simulink model "MATMPC_SIMULINK"  (R2017b)
settings: Solver=VariableStepAuto  StartTime=0.0  StopTime=4.0  RelTol=1e-3
values from neighbouring files (symbols this model uses):
  lb = 0*ones(nc,1)    [InitData.m]    (also in Initialization.m; Initialization_Simulink.m = 0)
  lbu = -80*ones(nu,1)    [InitData.m]    (also in InitData_ngrid.m = -inf(nu,1); Initialization.m; Initialization_Simulink.m = repmat(lbu,1,N))
  lbx = 0    [Initialization_Simulink.m]
  para = repmat(para0,1,N+1)    [InitData.m]    (also in InitData_ngrid.m = repmat(para0,1,r+1); Initialization.m; Initialization_Simulink.m)
  ref = zeros(ny,1)    [Initialization_Simulink.m]
  Ts = 0.2    [ChainofMasses_NLin.m]    (also in DiM.m = 0.01; InitData.m = settings.Ts; InitData_ngrid.m = settings.Ts; InitMemory.m = settings.Ts)
  ub = 12*ones(nc,1)    [InitData.m]    (also in Initialization.m; Initialization_Simulink.m = 0)
  ubu = 80*ones(nu,1)    [InitData.m]    (also in InitData_ngrid.m = inf(nu,1); Initialization.m; Initialization_Simulink.m = repmat(ubu,1,N))
  ubx = 0    [Initialization_Simulink.m]
  W = eye(3)    [DiM.m]    (also in Initialization_Simulink.m = diag([10 10 0.1 0.1 0.01]))
  WN = W(1:nyN,1:nyN)    [Initialization_Simulink.m]
  x0 = zeros(nx,1)    [InitData.m]    (also in Initialization.m; Initialization_Simulink.m = [0;pi;0;0])
settings Model: Creator=chen  LastModifiedBy=chen
settings RTWCC: CheckMdlBeforeBuild=Error

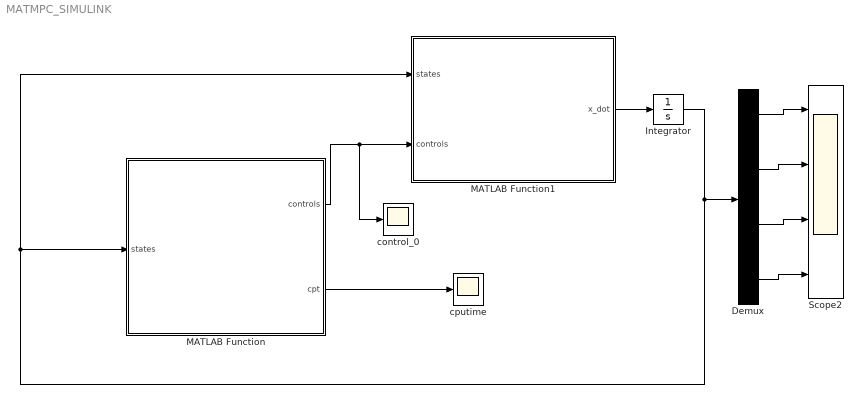
== system MATMPC_SIMULINK ==
  Demux : Demux
  Integrator : Integrator  InitialCondition=x0
  MATLAB Function : MATLAB Function  TreatAsAtomicUnit=on  SystemSampleTime=Ts
  MATLAB Function1 : MATLAB Function  TreatAsAtomicUnit=on
  Scope2 : Scope  NumInputPorts=4
  control_0 : Scope
  cputime : Scope
  wires:
  MATLAB Function/1(controls) -> control_0/1, MATLAB Function1/2(controls)
  MATLAB Function/2(cpt) -> cputime/1
  MATLAB Function1/1(x_dot) -> Integrator/1
  Integrator/1 -> Demux/1, MATLAB Function/1(states), MATLAB Function1/1(states)
  Demux/1 -> Scope2/1
  Demux/2 -> Scope2/2
  Demux/3 -> Scope2/3
  Demux/4 -> Scope2/4

== matlab function MATMPC_SIMULINK/MATLAB Function1 ==
  data: states input size=4; x_dot output size=4; controls input size=1
function x_dot  = Dynamics(states,controls)

M = 1; 
m = 0.1;
l = 0.8; 
g = 9.81;

p=states(1);
theta=states(2);
v=states(3);
omega=states(4);  
u=controls(1);

a=-m*l*sin(theta)*omega^2+m*g*cos(theta)*sin(theta)+u;
b=-m*l*cos(theta)*sin(theta)*omega^2+u*cos(theta)+(M+m)*g*sin(theta);
c=M+m-m*(cos(theta))^2;

x_dot = [v;omega;a/c;b/(l*c)];

return

== matlab function MATMPC_SIMULINK/MATLAB Function ==
  settings: updateMethod=DISCRETE
  data: states input size=4; controls output size=1; cpt output size=1; x0 parameter; lb parameter; ub parameter; lbx parameter; ubx parameter; lbu parameter; ubu parameter; W parameter; WN parameter; para parameter; ref parameter
function [controls,cpt] = NMPC_BLOCK(states, x0, lb, ub, lbx, ubx, lbu, ubu, W, WN, para, ref)

%% everything should has a fixed size

coder.extrinsic('mpc_nmpcsolver_simulink');  
coder.extrinsic('InitData');  
coder.extrinsic('InitMemory');  
%%

persistent x u lambda mu mu_x mu_u;
persistent input mem opt settings;

if isempty(x)  
    
    N=40;
    N2=5;
    Ts  = 0.05;
    Ts_st = 0.05;
    s = 2;     
    nx = 4;    
    nu = 1;   
    ny = 5;    
    nyN= 4;   
    np = 0;    
    nc = 0;    
    ncN = 0;  
    nbx = 1;
    nbu = 1;
    nbu_idx = 1;
    nbx_idx = 1;
    
    settings.N=N;
    settings.N2=N2;
    settings.Ts = Ts;
    settings.Ts_st = Ts_st;
    settings.s =s ;
    settings.nx = nx; 
    settings.nu = nu;    
    settings.ny = ny;    
    settings.nyN= nyN;    
    settings.np = np;   
    settings.nc = nc;
    settings.ncN = ncN;
    settings.nbx = nbx;
    settings.nbu = nbu;
    settings.nbx_idx = nbx_idx;
    settings.nbu_idx = nbu_idx;
    settings.model='InvertedPendulum';
    
    opt.integrator='ERK4-CASADI'; % 'ERK4','IRK3, 'ERK4-CASADI'
    opt.hessian='gauss_newton';  % 'gauss_newton'
    opt.condensing='default_full';  %'default_full','no'
    opt.qpsolver='qpoases'; %'qpoases','qore', 'quadprog', 'hpipm_sparse', 'hpipm_pcond'
    opt.hotstart='no'; %'yes','no' (only for qpoases)
    opt.shifting='yes'; % 'yes','no'
    opt.lin_obj='yes'; % 'yes','no' % if objective function is linear least square
    opt.ref_type=0; % 0-time invariant, 1-time varying(no preview), 2-time varying (preview)
   
    input.x0=x0;
    
    x=repmat(x0,1,N+1);
    input.x=x;
    
    u=zeros(nu,N);
    input.u=u;
    
    lambda = zeros(nx,N+1);
    input.lambda= lambda;
    
    if N*nc+ncN > 0
        mu = zeros(N*nc+ncN,1);
    else
        mu = 0;
    end
    input.mu= mu;
    
    mu_u = zeros(N*nu,1);
    input.mu_u= mu_u;
    
    if (N+1)*nbx > 0
        mu_x = zeros((N+1)*nbx,1);
    else
        mu_x = 0;
    end
    input.mu_x = mu_x;
    
    input.lb = lb;
    input.ub = ub;
    input.lbx = lbx;
    input.ubx = ubx;
    input.lbu = lbu;
    input.ubu = ubu;
    
    input.W=W;
    input.WN=WN;
    input.od = para;
    
    input.y = repmat(ref,1,N);
    input.yN = ref(1:nyN,1);
    
    mem.warm_start=0;
    mem.hot_start=0;
    if strcmp(opt.hotstart, 'yes')
        mem.hot_start=1;
    end
    
    mem.qpoases_opt = qpOASES_options('MPC');
     
    mem.mu0=1e2;
    mem.max_qp_it = 100;
    mem.pred_corr = 1;
    mem.cond_pred_corr = 1;

    mem.qore_id = -1;
    
    mem.sim_method = 0;
    
    mem.sqp_maxit = 1;           % maximum number of iterations for each sampling instant (for RTI, this is ONE)
    mem.kkt_lim = 1e-1;          % tolerance on optimality
    mem.mu_merit=0;              % initialize the parameter
    mem.eta=1e-4;                % merit function parameter
    mem.tau=0.8;                 % step length damping factor
    mem.mu_safty=1.1;            % constraint weight update factor (for merit function)
    mem.rho=0.5;                 % merit function parameter
    
    mem.A = zeros(nx,nx*N);
    mem.B = zeros(nx,nu*N);
    mem.Cx = zeros(nbx,nx);
    mem.Cgx = zeros(nc,nx*N);
    mem.Cgu = zeros(nc,nu*N);
    mem.CgN = zeros(ncN,nx);
    mem.gx = zeros(nx,N+1);
    mem.gu = zeros(nu,N);
    mem.a = zeros(nx,N);
    mem.ds0 = zeros(nx,1);
    mem.lc = zeros(N*nc+ncN,1);
    mem.uc = zeros(N*nc+ncN,1);
    mem.lb_du = zeros(N*nu,1);
    mem.ub_du = zeros(N*nu,1);
    mem.lb_dx = zeros((N+1)*nbx,1);
    mem.ub_dx = zeros((N+1)*nbx,1);
    
    mem.Hc = zeros(N*nu,N*nu);
    mem.Ccx = zeros((N+1)*nbx,N*nu);
    mem.Ccg = zeros(N*nc+ncN,N*nu);
    mem.gc = zeros(N*nu,1);
    mem.lcc = zeros(N*nc+ncN,1);
    mem.ucc = zeros(N*nc+ncN,1);
    mem.lxc = zeros((N+1)*nbx,1);
    mem.uxc = zeros((N+1)*nbx,1);
    
    mem.dx = zeros(nx,N+1);
    mem.du = zeros(nu,N);
    mem.lambda_new = zeros(nx,N+1);
    mem.mu_new = zeros(N*nc+ncN,1);
    mem.mu_x_new = zeros((N+1)*nbx,1);
    mem.mu_u_new = zeros(N*nu,1);
    
    for i=1:nbx
        mem.Cx(i,nbx_idx(i)) = 1.0;
    end
    
    mem.lin_obj = 0;    
    mem.Q = zeros(nx,nx*(N+1));
    mem.S = zeros(nx,nu*N);
    mem.R = zeros(nu,nu*N);
   
    mem.reg = 1e-8;   
    mem.iter=1;
             
else
    %Update the component of mem that changed

    input.x=x; 
    input.u=u;
    input.lambda=lambda;   
    input.mu=mu;
    input.mu_x=mu_x;
    input.mu_u=mu_u;
    
end

%%
input.x0 = states;

cpt = 0;
[input,mem,cpt]=mpc_nmpcsolver_simulink(input, settings, mem, opt);

controls = input.u(1,1);

%% shift by hand!
switch opt.shifting
    case 'yes'
        x=[input.x(:,2:end),input.x(:,end)];  
        u=[input.u(:,2:end),input.u(:,end)]; 
        lambda=[input.lambda(:,2:end),input.lambda(:,end)];
%        mu=[input.mu(nc+1:N*nc+ncN,1);input.mu(N*nc+ncN-nc+1:N*nc+ncN,1)];
        mu_x=[input.mu_x(2:end,1);input.mu_x(end,1)];
        mu_u=[input.mu_u(2:end,1);input.mu_u(end,1)];
   case 'no'
        x=input.x;
        u=input.u;
        lambda=input.lambda;
        mu=input.mu;
        mu_x=input.mu_x;
        mu_u=input.mu_u;
end

return
